simulink model "EKF_SImulink_Ass_3"  (R2024b)
settings: Solver=VariableStepAuto  StartTime=0.0  StopTime=tf  RelTol=1e-3
values from neighbouring files (symbols this model uses):
  C = [1,0,0,0 ... (first row only)    [main.m]
  IC = [0;0; 0; 0]    [main.m]
  Qk = eye(2)    [main.m]
  Rk = [1,0;0,1]    [main.m]
  Wamp = 2    [main.m]
settings Model: Creator=anton  LastModifiedBy=gabri

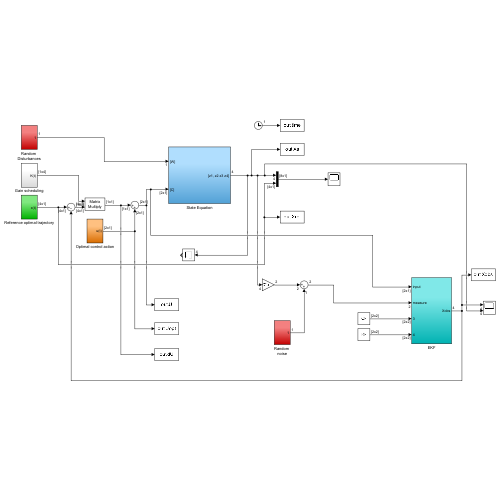
[thumbnail: Simulink's stored preview of the top-level diagram]
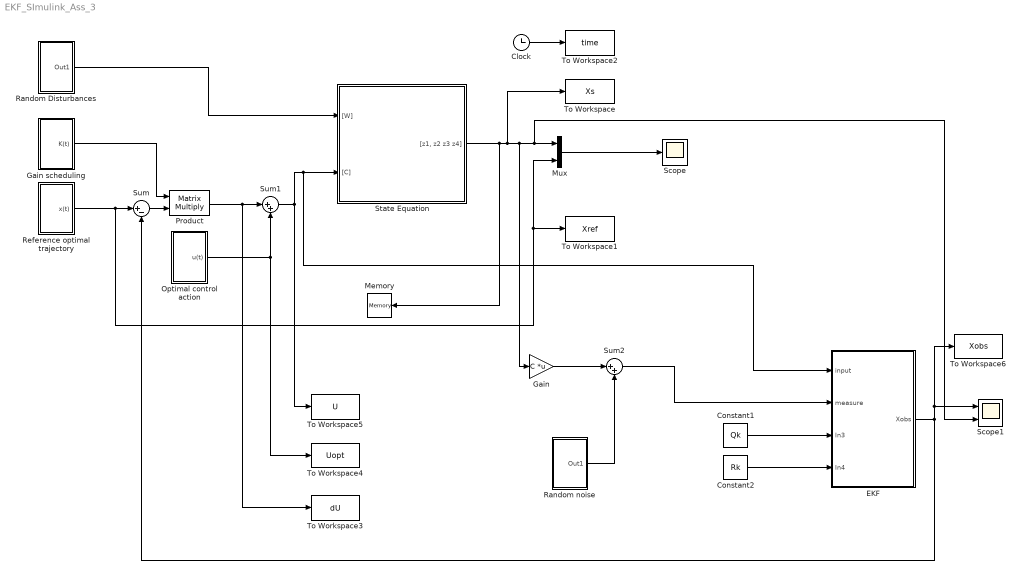
== system EKF_SImulink_Ass_3 ==
  Clock : Clock
  Constant1 : Constant  Value=Qk
  Constant2 : Constant  Value=Rk
  EKF : Subsystem
  Gain : Gain  Gain=C  Multiplication=Matrix(K*u)
  Gain scheduling : Subsystem
  Memory : Memory
  Mux : Mux  Inputs=2
  Optimal control action : Subsystem
  Product : Product  Multiplication=Matrix(*)
  Random Disturbances : Subsystem
  Random noise : Subsystem
  Reference optimal trajectory : Subsystem
  Scope : Scope
  Scope1 : Scope  NumInputPorts=2
  State Equation : Subsystem
  Sum : Sum  Inputs=|+-
  Sum1 : Sum  Inputs=|++
  Sum2 : Sum  Inputs=|++
  To Workspace : ToWorkspace  VariableName=Xs  SaveFormat=Timeseries  SampleTime=-1
  To Workspace1 : ToWorkspace  VariableName=Xref  SaveFormat=Timeseries  SampleTime=-1
  To Workspace2 : ToWorkspace  VariableName=time  SaveFormat=Timeseries  SampleTime=-1
  To Workspace3 : ToWorkspace  VariableName=dU  SaveFormat=Timeseries  SampleTime=-1
  To Workspace4 : ToWorkspace  VariableName=Uopt  SaveFormat=Timeseries  SampleTime=-1
  To Workspace5 : ToWorkspace  VariableName=U  SaveFormat=Timeseries  SampleTime=-1
  To Workspace6 : ToWorkspace  VariableName=Xobs  SaveFormat=Timeseries  SampleTime=-1
  wires:
  Reference optimal trajectory/1(x(t)) -> To Workspace1/1, Mux/2, Sum/1
  Optimal control action/1(u(t)) -> To Workspace4/1, Sum1/2
  Clock/1 -> To Workspace2/1
  Sum/1 -> Product/2
  Sum1/1 -> To Workspace5/1, EKF/1(input), State Equation/2("[C]")
  Gain scheduling/1(K(t)) -> Product/1
  State Equation/1("[z1, z2 z3 z4]") -> To Workspace/1, Gain/1, Scope1/2, Mux/1, Memory/1
  Mux/1 -> Scope/1
  Random Disturbances/1(Out1) -> State Equation/1("[W]")
  Product/1 -> Sum1/1, To Workspace3/1
  Gain/1 -> Sum2/1
  Random noise/1(Out1) -> Sum2/2
  Constant2/1 -> EKF/4(In4)
  Sum2/1 -> EKF/2(measure)
  Constant1/1 -> EKF/3(In3)
  EKF/1(Xobs) -> Sum/2, To Workspace6/1, Scope1/1

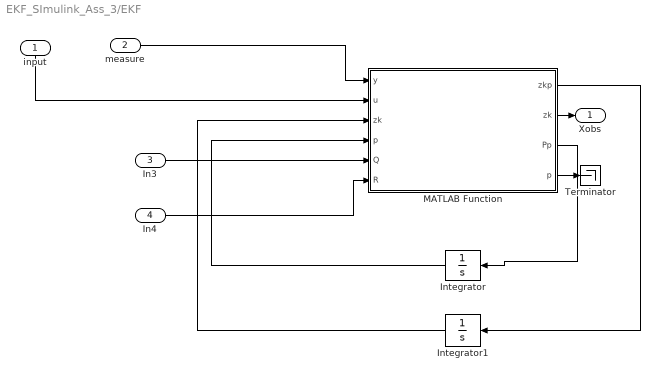
== system EKF_SImulink_Ass_3/EKF ==
  input : Inport
  measure : Inport  Port=2
  In3 : Inport  Port=3
  In4 : Inport  Port=4
  Integrator : Integrator  InitialCondition=zeros(16,1)
  Integrator1 : Integrator  InitialCondition=IC
  MATLAB Function : MATLAB Function  TreatAsAtomicUnit=on
  Terminator : Terminator
  Xobs : Outport
  wires:
  MATLAB Function/1(zkp) -> Integrator1/1
  Integrator1/1 -> MATLAB Function/3("zk ")
  MATLAB Function/2(zk) -> Xobs/1
  MATLAB Function/4(p) -> Terminator/1
  input/1 -> MATLAB Function/2(u)
  In4/1 -> MATLAB Function/6(R)
  Integrator/1 -> MATLAB Function/4("p ")
  In3/1 -> MATLAB Function/5(Q)
  measure/1 -> MATLAB Function/1(y)
  MATLAB Function/3(Pp) -> Integrator/1

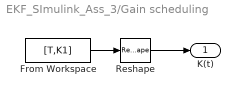
== system EKF_SImulink_Ass_3/Gain scheduling ==
  From Workspace : FromWorkspace  VariableName=[T,K1]
  Reshape : Reshape  OutputDimensionality=Row vector (2-D)
  K(t) : Outport
  wires:
  From Workspace/1 -> Reshape/1
  Reshape/1 -> K(t)/1

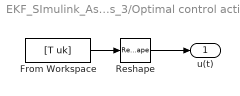
== system EKF_SImulink_Ass_3/Optimal control action ==
  From Workspace : FromWorkspace  VariableName=[T uk]
  Reshape : Reshape  OutputDimensionality=Column vector (2-D)
  u(t) : Outport
  wires:
  From Workspace/1 -> Reshape/1
  Reshape/1 -> u(t)/1

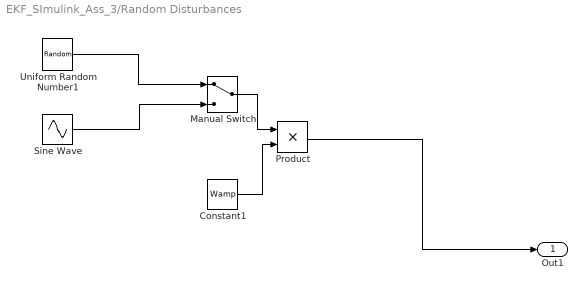
== system EKF_SImulink_Ass_3/Random Disturbances ==
  Constant1 : Constant  Value=Wamp
  Manual Switch : ManualSwitch
  Product : Product
  Sine Wave : Sin  Frequency=2*pi*100  SampleTime=0
  Uniform Random Number1 : UniformRandomNumber  SampleTime=tf/1000
  Out1 : Outport
  wires:
  Product/1 -> Out1/1
  Constant1/1 -> Product/2
  Uniform Random Number1/1 -> Manual Switch/1
  Sine Wave/1 -> Manual Switch/2
  Manual Switch/1 -> Product/1

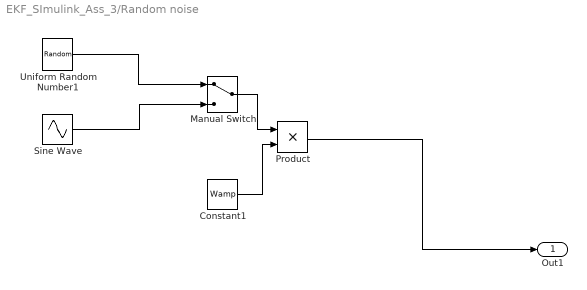
== system EKF_SImulink_Ass_3/Random noise ==
  Constant1 : Constant  Value=Wamp
  Manual Switch : ManualSwitch
  Product : Product
  Sine Wave : Sin  Frequency=2*pi*100  SampleTime=0
  Uniform Random Number1 : UniformRandomNumber  SampleTime=tf/1000
  Out1 : Outport
  wires:
  Manual Switch/1 -> Product/1
  Sine Wave/1 -> Manual Switch/2
  Uniform Random Number1/1 -> Manual Switch/1
  Constant1/1 -> Product/2
  Product/1 -> Out1/1

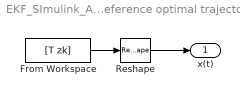
== system EKF_SImulink_Ass_3/Reference optimal trajectory ==
  From Workspace : FromWorkspace  VariableName=[T zk]
  Reshape : Reshape  OutputDimensionality=Column vector (2-D)
  x(t) : Outport
  wires:
  From Workspace/1 -> Reshape/1
  Reshape/1 -> x(t)/1

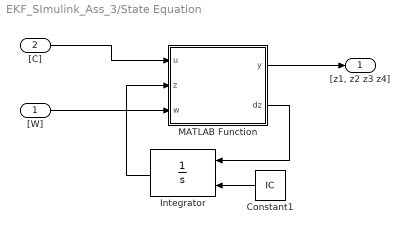
== system EKF_SImulink_Ass_3/State Equation ==
  "[W]" : Inport
  "[C]" : Inport  Port=2
  Constant1 : Constant  Value=IC
  Integrator : Integrator  InitialConditionSource=external
  MATLAB Function : MATLAB Function  TreatAsAtomicUnit=on
  "[z1, z2 z3 z4]" : Outport
  wires:
  MATLAB Function/2(dz) -> Integrator/1
  Integrator/1 -> MATLAB Function/2(z)
  Constant1/1 -> Integrator/2
  MATLAB Function/1(y) -> "[z1, z2 z3 z4]"/1
  "[C]"/1 -> MATLAB Function/1(u)
  "[W]"/1 -> MATLAB Function/3(w)

== matlab function EKF_SImulink_Ass_3/EKF/MATLAB Function ==
  data: y input; u input; zkp output; zk input; zk output; Pp output; p output; p input; Q input; R input
function [zkp,zk,Pp,p]  = obs(y,u,zk,p,Q,R)

Nstates = size(zk,1);

zkp = zeros(Nstates,1);
Pp = zeros(Nstates^2,1);

% Data of the pendulum
g = 9.81; % [m/s^2] gravity
m   = 1;          % massa del corpo [kg]
Cd  = 0.15;       % coefficiente di resistenza aerodinamica (attrito quadratico)
epsilon = 1;
mu_r = 1;
%% Linearization around the estimated position A,C,L

% Jacobian of the dynamics
A = [0 0 -zk(4)*sin(zk(3))  cos(zk(3));
         0 0  zk(4)*cos(zk(3))  sin(zk(3));
         0 0  0           0;
         0 0  0       -2*Cd*zk(4)/m-(mu_r*9.81)/(cosh(zk(4)/epsilon)^2*epsilon)];

Lm = [0 0;
      0 0;
      0 1; 
      1/m 0];

% observation matrix
C = [1,0,0,0;
    0,1,0,0];

%% Differential Riccati Equation - Computation of the gain matrix K

% transformation vector -> matrix
P = zeros(Nstates,Nstates);
P(1:end) = p(1:end,1);

% DRE
Out = (A*P + P*A' + Lm*Q*Lm' - P*C'*R^-1*C*P);

K = P*C'*R^-1;

% transformation matrix -> vector
Pp(1:end,1) = Out(1:end)';

%% State estimate

zkp(:,1) = [ zk(4)*cos(zk(3));  zk(4)*sin(zk(3)) ;  u(2);    1/m*(u(1) - Cd*zk(4)^2 - mu_r*m*9.81*tanh(zk(4)/epsilon))];          

zkp = zkp + K*(y - C*zk);

== matlab function EKF_SImulink_Ass_3/State Equation/MATLAB Function ==
  data: u input; z input; w input; y output; dz output
% function [y,dx]  = fcn(c,w,x)
% 
% m = 1;
% g = 9.81;
% L = 0.1;
% zeta = 0.02;
% w0 = sqrt(g/L);
% 
% dx = zeros(2,1);
% 
% u = c + w;
% 
% dx(1) = - 2*zeta*w0*x(1) - w0^2*sin(x(2)) + u/L^2/m;
% dx(2) = x(1);
% 
% y = [x(1);x(2)];


function [y, dz] = stateEq_new(u,z,w)

%% ========================================================================
% Funzione: stateEq_new
% ------------------------------------------------------------------------
% Descrizione:
%   Definisce le equazioni di stato del sistema dinamico non lineare.
%   Lo stato è composto da:
%       z = [x; y; θ; v]
%   dove:
%       x, y  → posizione
%       θ     → orientamento
%       v     → velocità
%   I controlli sono:
%       u1 → forza di trazione (accelerazione lungo la direzione θ)
%       u2 → controllo di rotazione (variazione dell'angolo θ)
%   Il modello include una resistenza aerodinamica proporzionale a v².
%
%   Equazioni:
%       ẋ = v*cos(θ)
%       ẏ = v*sin(θ)
%       θ̇ = u2
%       v̇ = (1/m)*(u1 - Cd*v²)
%
% Input:
%   t   → tempo corrente
%   z   → stato corrente [x; y; θ; v]
%   u   → controllo definito sulla griglia temporale Tu
%   Tu  → vettore temporale del controllo
%   m   → massa
%   Cd  → coefficiente di resistenza aerodinamica
%   w   → disturbo esterno
%
% Output:
%   dz  → derivata dello stato (vettore 4x1)
%% ========================================================================

    m   = 1;          % massa del corpo [kg]
    Cd  = 0.15;       % coefficiente di resistenza aerodinamica (attrito quadratico)
    mu_r = 1;
    epsilon = 1;

    dz = zeros(4,1);                     % inizializza derivata stato

    % Interpolazione dei controlli u1(t) e u2(t) al tempo corrente t
    u1 = u(1) + w;
    u2 = u(2) + w;

    % Equazioni dinamiche del sistema
    dz(1) = z(4)*cos(z(3));              % ẋ = v * cos(θ)
    dz(2) = z(4)*sin(z(3));              % ẏ = v * sin(θ)
    dz(3) = u2;                          % θ̇ = u2 (velocità angolare)
    dz(4) = 1/m*(u1 - Cd*z(4)^2      - mu_r*m*9.81*tanh(z(4)/epsilon));        % v̇ = (u1 - Cd*v²)/m

    y = [z(1); z(2); z(3); z(4)];

end
